simulink model "model_podstawowy_2018b"  (R2018b)
settings: Solver=VariableStepAuto  StartTime=0.0  StopTime=15  RelTol=1e-3
undefined symbols (not defined in the file): g, J, K_reg, L, m, M, Q2, x_konc, x_pocz
settings Model: Creator=maelstro  LastModifiedBy=maelstro
settings DataIOCC: ReturnWorkspaceOutputs=on

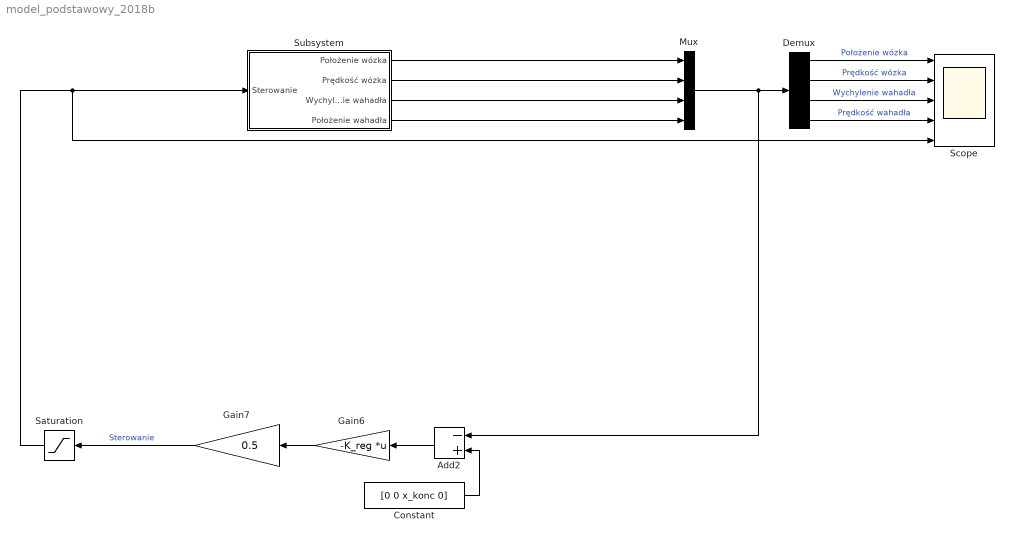
== system model_podstawowy_2018b ==
  Add2 : Sum  Inputs=-+
  Constant : Constant  Value=[0 0 x_konc 0]
  Demux : Demux
  Gain6 : Gain  Gain=-K_reg  Multiplication=Matrix(K*u)
  Gain7 : Gain  Gain=0.5
  Mux : Mux
  Saturation : Saturate  UpperLimit=6  LowerLimit=-6
  Scope : Scope  NumInputPorts=5
  Subsystem : Subsystem
  wires:
  Gain6/1 -> Gain7/1
  Add2/1 -> Gain6/1
  Mux/1 -> Demux/1, Add2/1
  Constant/1 -> Add2/2
  Subsystem/1(Położenie wózka) -> Mux/1
  Subsystem/2(Prędkość wózka) -> Mux/2
  Subsystem/3(Wychylenie wahadła) -> Mux/3
  Subsystem/4(Położenie wahadła) -> Mux/4
  Demux/1 -> Scope/1  "Położenie wózka"
  Demux/2 -> Scope/2  "Prędkość wózka"
  Demux/3 -> Scope/3  "Wychylenie wahadła"
  Demux/4 -> Scope/4  "Prędkość wahadła"
  Gain7/1 -> Saturation/1  "Sterowanie"
  Saturation/1 -> Scope/5, Subsystem/1(Sterowanie)

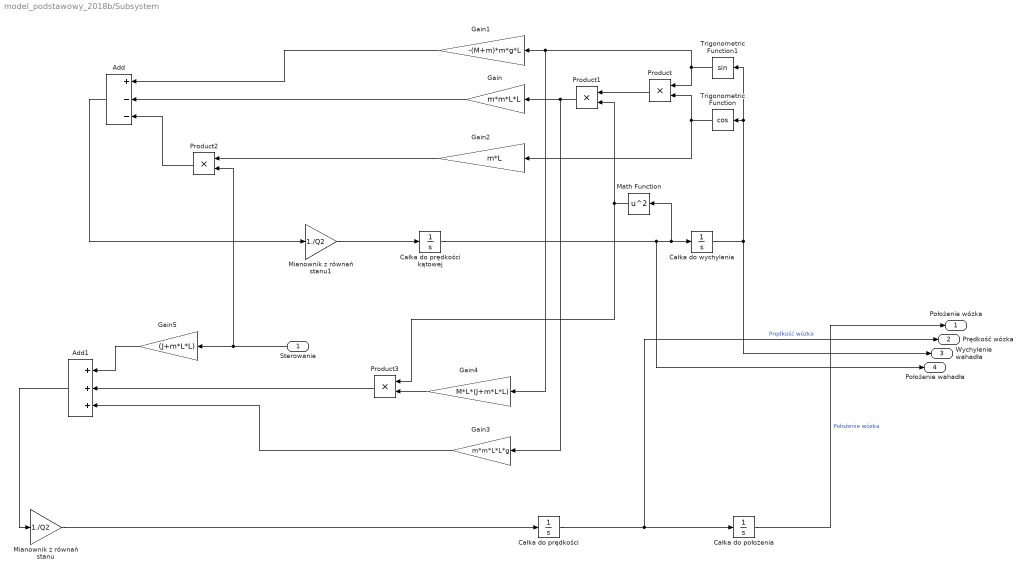
== system model_podstawowy_2018b/Subsystem ==
  Sterowanie : Inport
  Add : Sum  Inputs=+--
  Add1 : Sum  Inputs=+++
  Całka do położenia : Integrator
  Całka do prędkości : Integrator
  Całka do prędkości kątowej : Integrator
  Całka do wychylenia : Integrator  InitialCondition=x_pocz
  Gain : Gain  Gain=m*m*L*L
  Gain1 : Gain  Gain=-(M+m)*m*g*L
  Gain2 : Gain  Gain=m*L
  Gain3 : Gain  Gain=m*m*L*L*g
  Gain4 : Gain  Gain=M*L*(J+m*L*L)
  Gain5 : Gain  Gain=(J+m*L*L)
  Math Function : Math  Operator=square  SaturateOnIntegerOverflow=on
  Mianownik z równań stanu : Gain  Gain=1./Q2
  Mianownik z równań stanu1 : Gain  Gain=1./Q2
  Product{,1..3} (4 alike) : Product
  Trigonometric Function : Trigonometry  Operator=cos
  Trigonometric Function1 : Trigonometry
  Położenie wózka : Outport
  Prędkość wózka : Outport  Port=2
  Wychylenie wahadła : Outport  Port=3
  Położenie wahadła : Outport  Port=4
  wires:
  Add1/1 -> Mianownik z równań stanu/1
  Add/1 -> Mianownik z równań stanu1/1
  Całka do prędkości/1 -> Prędkość wózka/1, Całka do położenia/1  "Prędkość wózka"
  Math Function/1 -> Product1/2, Product3/1
  Gain4/1 -> Product3/2
  Sterowanie/1 -> Product2/2, Gain5/1
  Product3/1 -> Add1/2
  Trigonometric Function/1 -> Gain2/1, Product/2
  Gain2/1 -> Product2/1
  Product1/1 -> Gain/1, Gain3/1
  Całka do wychylenia/1 -> Wychylenie wahadła/1, Trigonometric Function1/1, Trigonometric Function/1
  Całka do położenia/1 -> Położenie wózka/1  "Położenie wózka"
  Mianownik z równań stanu/1 -> Całka do prędkości/1
  Trigonometric Function1/1 -> Product/1, Gain4/1, Gain1/1
  Mianownik z równań stanu1/1 -> Całka do prędkości kątowej/1
  Gain/1 -> Add/2
  Gain1/1 -> Add/1
  Product/1 -> Product1/1
  Product2/1 -> Add/3
  Gain3/1 -> Add1/3
  Całka do prędkości kątowej/1 -> Położenie wahadła/1, Math Function/1, Całka do wychylenia/1
  Gain5/1 -> Add1/1
